simulink model "PulsePairProc"  (Simulink 6.4)
settings: Solver=ode45  StartTime=0.0  StopTime=40000/12e6  RelTol=1e-3
libraries: xbsIndex_r4 x256, simulink x2, dspsrcs4 x1
(part 1 of 2)
settings Model: LastModifiedBy=tbrimeye

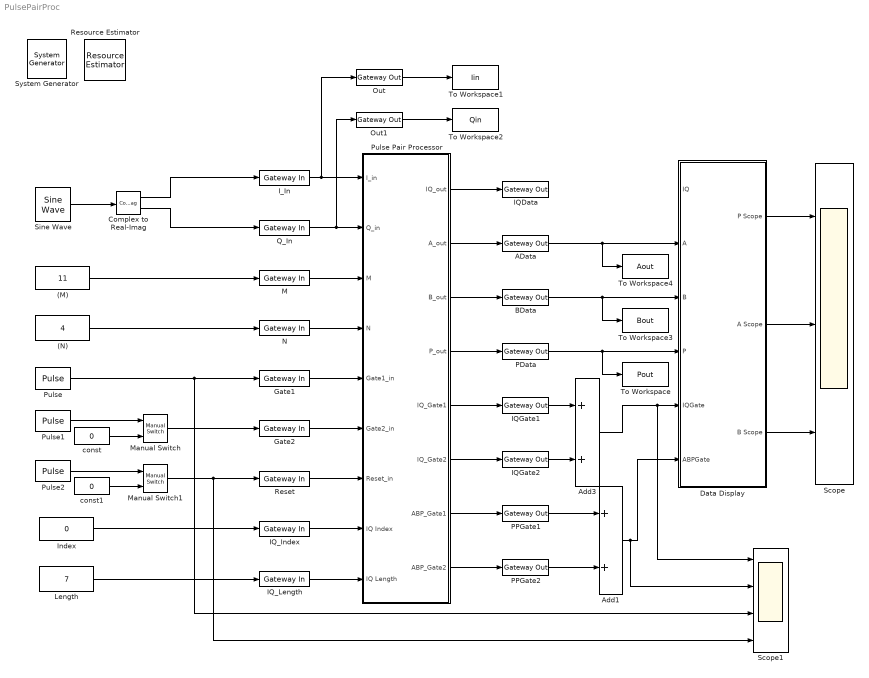
== system PulsePairProc ==
  " System Generator" : xbsIndex_r4/ System Generator  Tag=genX  SystemSampleTime=-1  xilinxfamily=Virtex4  part=xc4vlx60  speed=-11  package=ff668  synthesis_tool=XST  directory=C:/Work_Projects/Xilinx/SysGen_Outputs/PulsePairProcessor/PulsePairProc_x1_netlist  testbench=off  simulink_period=1/12e6  sysclk_period=(1/12e6)*1e9  incr_netlist=off  trim_vbits=Everywhere in SubSystem  dbl_ovrd=According to Block Masks  core_generation=According to Block Masks  run_coregen=off  deprecated_control=off  eval_field=0  block_type=sysgen
      settings: block_version=8.2
  (M) : Constant  Value=11  OutDataType=sfix(16)  ConRadixGroup=Use specified scaling  OutScaling=2^0  SampleTime=inf  FramePeriod=inf
  (N) : Constant  Value=4  OutDataType=sfix(16)  ConRadixGroup=Use specified scaling  OutScaling=2^0  SampleTime=inf  FramePeriod=inf
  AData : xbsIndex_r4/Gateway Out  hdl_port=on  timing_constraint=None  locs_specified=off  LOCs={}  block_type=gatewayout
      settings: infoedit="Gateway out block.  Converts Xilinx fixed point inputs into ouputs of type Simulink integer, double, or fixed point.<P><P>Hardware notes:  In hardware these blocks become top level output ports or are discarded, depending on how they are configured."  xl_area=[0 0 0 0 32 0 0]  block_version=8.2
  Add1 : Sum  OutScaling=2^-10
  Add3 : Sum  OutScaling=2^-10
  BData : xbsIndex_r4/Gateway Out  hdl_port=on  timing_constraint=None  locs_specified=off  LOCs={}  block_type=gatewayout
      settings: infoedit="Gateway out block.  Converts Xilinx fixed point inputs into ouputs of type Simulink integer, double, or fixed point.<P><P>Hardware notes:  In hardware these blocks become top level output ports or are discarded, depending on how they are configured."  xl_area=[0 0 0 0 32 0 0]  block_version=8.2
  Complex to Real-Imag : ComplexToRealImag
  Data Display : Subsystem
  Gate1 : xbsIndex_r4/Gateway In  arith_type=Boolean  n_bits=18  bin_pt=0  quantization="Round  (unbiased: +/- Inf)"  overflow=Flag as error  period=1/12e6  dbl_ovrd=off  timing_constraint=None  locs_specified=off  LOCs={}  block_type=gatewayin
      settings: infoedit="Gateway in block.  Converts inputs of type Simulink integer, double and fixed point to  Xilinx fixed point type.<P><P>Hardware notes:  In hardware these blocks become top level input ports."  xl_area=[0 0 0 0 1 0 0]  block_version=8.2
  Gate2 : xbsIndex_r4/Gateway In  arith_type=Boolean  n_bits=18  bin_pt=0  quantization="Round  (unbiased: +/- Inf)"  overflow=Flag as error  period=1/12e6  dbl_ovrd=off  timing_constraint=None  locs_specified=off  LOCs={}  block_type=gatewayin
      settings: infoedit="Gateway in block.  Converts inputs of type Simulink integer, double and fixed point to  Xilinx fixed point type.<P><P>Hardware notes:  In hardware these blocks become top level input ports."  xl_area=[0 0 0 0 1 0 0]  block_version=8.2
  IQData : xbsIndex_r4/Gateway Out  hdl_port=on  timing_constraint=None  locs_specified=off  LOCs={}  block_type=gatewayout
      settings: infoedit="Gateway out block.  Converts Xilinx fixed point inputs into ouputs of type Simulink integer, double, or fixed point.<P><P>Hardware notes:  In hardware these blocks become top level output ports or are discarded, depending on how they are configured."  xl_area=[0 0 0 0 32 0 0]  block_version=8.2
  IQGate1 : xbsIndex_r4/Gateway Out  hdl_port=on  timing_constraint=None  locs_specified=off  LOCs={}  block_type=gatewayout
      settings: infoedit="Gateway out block.  Converts Xilinx fixed point inputs into ouputs of type Simulink integer, double, or fixed point.<P><P>Hardware notes:  In hardware these blocks become top level output ports or are discarded, depending on how they are configured."  xl_area=[0 0 0 0 1 0 0]  block_version=8.2
  IQGate2 : xbsIndex_r4/Gateway Out  hdl_port=on  timing_constraint=None  locs_specified=off  LOCs={}  block_type=gatewayout
      settings: infoedit="Gateway out block.  Converts Xilinx fixed point inputs into ouputs of type Simulink integer, double, or fixed point.<P><P>Hardware notes:  In hardware these blocks become top level output ports or are discarded, depending on how they are configured."  xl_area=[0 0 0 0 1 0 0]  block_version=8.2
  IQ_Index : xbsIndex_r4/Gateway In  arith_type=Unsigned  n_bits=10  bin_pt=0  quantization="Round  (unbiased: +/- Inf)"  overflow=Flag as error  period=1/12e6  dbl_ovrd=off  timing_constraint=None  locs_specified=off  LOCs={}  block_type=gatewayin
      settings: infoedit="Gateway in block.  Converts inputs of type Simulink integer, double and fixed point to  Xilinx fixed point type.<P><P>Hardware notes:  In hardware these blocks become top level input ports."  xl_area=[0 0 0 0 10 0 0]  block_version=8.2
  IQ_Length : xbsIndex_r4/Gateway In  arith_type=Unsigned  n_bits=10  bin_pt=0  quantization="Round  (unbiased: +/- Inf)"  overflow=Flag as error  period=1/12e6  dbl_ovrd=off  timing_constraint=None  locs_specified=off  LOCs={}  block_type=gatewayin
      settings: infoedit="Gateway in block.  Converts inputs of type Simulink integer, double and fixed point to  Xilinx fixed point type.<P><P>Hardware notes:  In hardware these blocks become top level input ports."  xl_area=[0 0 0 0 10 0 0]  block_version=8.2
  I_In : xbsIndex_r4/Gateway In  arith_type="Signed  (2's comp)"  n_bits=16  bin_pt=15  quantization="Round  (unbiased: +/- Inf)"  overflow=Saturate  period=1/12e6  dbl_ovrd=off  timing_constraint=None  locs_specified=off  LOCs={}  block_type=gatewayin
      settings: infoedit="Gateway in block.  Converts inputs of type Simulink integer, double and fixed point to  Xilinx fixed point type.<P><P>Hardware notes:  In hardware these blocks become top level input ports."  xl_area=[0 0 0 0 16 0 0]  block_version=8.2
  Index : Constant  Value=0  OutDataType=sfix(16)  ConRadixGroup=Use specified scaling  OutScaling=2^0  SampleTime=inf  FramePeriod=inf
  Length : Constant  Value=7  OutDataType=sfix(16)  ConRadixGroup=Use specified scaling  OutScaling=2^0  SampleTime=inf  FramePeriod=inf
  M : xbsIndex_r4/Gateway In  arith_type=Unsigned  n_bits=11  bin_pt=0  quantization="Round  (unbiased: +/- Inf)"  overflow=Flag as error  period=1/12e6  dbl_ovrd=off  timing_constraint=None  locs_specified=off  LOCs={}  block_type=gatewayin
      settings: infoedit="Gateway in block.  Converts inputs of type Simulink integer, double and fixed point to  Xilinx fixed point type.<P><P>Hardware notes:  In hardware these blocks become top level input ports."  xl_area=[0 0 0 0 11 0 0]  block_version=8.2
  Manual Switch : simulink/Signal Routing/Manual Switch  SystemSampleTime=-1  sw=0  action=0
  Manual Switch1 : simulink/Signal Routing/Manual Switch  SystemSampleTime=-1  sw=1  action=0
  N : xbsIndex_r4/Gateway In  arith_type=Unsigned  n_bits=7  bin_pt=0  quantization="Round  (unbiased: +/- Inf)"  overflow=Flag as error  period=1/12e6  dbl_ovrd=off  timing_constraint=None  locs_specified=off  LOCs={}  block_type=gatewayin
      settings: infoedit="Gateway in block.  Converts inputs of type Simulink integer, double and fixed point to  Xilinx fixed point type.<P><P>Hardware notes:  In hardware these blocks become top level input ports."  xl_area=[0 0 0 0 7 0 0]  block_version=8.2
  Out : xbsIndex_r4/Gateway Out  hdl_port=off  timing_constraint=None  locs_specified=off  LOCs={}  block_type=gatewayout
      settings: infoedit="Gateway out block.  Converts Xilinx fixed point inputs into ouputs of type Simulink integer, double, or fixed point.<P><P>Hardware notes:  In hardware these blocks become top level output ports or are discarded, depending on how they are configured."  xl_area=[0 0 0 0 0 0 0]  block_version=8.2
  Out1 : xbsIndex_r4/Gateway Out  hdl_port=off  timing_constraint=None  locs_specified=off  LOCs={}  block_type=gatewayout
      settings: infoedit="Gateway out block.  Converts Xilinx fixed point inputs into ouputs of type Simulink integer, double, or fixed point.<P><P>Hardware notes:  In hardware these blocks become top level output ports or are discarded, depending on how they are configured."  xl_area=[0 0 0 0 0 0 0]  block_version=8.2
  PData : xbsIndex_r4/Gateway Out  hdl_port=on  timing_constraint=None  locs_specified=off  LOCs={}  block_type=gatewayout
      settings: infoedit="Gateway out block.  Converts Xilinx fixed point inputs into ouputs of type Simulink integer, double, or fixed point.<P><P>Hardware notes:  In hardware these blocks become top level output ports or are discarded, depending on how they are configured."  xl_area=[0 0 0 0 32 0 0]  block_version=8.2
  PPGate1 : xbsIndex_r4/Gateway Out  hdl_port=on  timing_constraint=None  locs_specified=off  LOCs={}  block_type=gatewayout
      settings: infoedit="Gateway out block.  Converts Xilinx fixed point inputs into ouputs of type Simulink integer, double, or fixed point.<P><P>Hardware notes:  In hardware these blocks become top level output ports or are discarded, depending on how they are configured."  xl_area=[0 0 0 0 1 0 0]  block_version=8.2
  PPGate2 : xbsIndex_r4/Gateway Out  hdl_port=on  timing_constraint=None  locs_specified=off  LOCs={}  block_type=gatewayout
      settings: infoedit="Gateway out block.  Converts Xilinx fixed point inputs into ouputs of type Simulink integer, double, or fixed point.<P><P>Hardware notes:  In hardware these blocks become top level output ports or are discarded, depending on how they are configured."  xl_area=[0 0 0 0 1 0 0]  block_version=8.2
  Pulse : DiscretePulseGenerator  PulseType=Time based  Period=22/12e6  PulseWidth=50  PhaseDelay=20/12e6
  Pulse Pair Processor : Subsystem
  Pulse1 : DiscretePulseGenerator  PulseType=Time based  Period=900/40e6  PulseWidth=10  PhaseDelay=150/12e6
  Pulse2 : DiscretePulseGenerator  PulseType=Time based  Period=500/12e6  PhaseDelay=10/12e6
  Q_In : xbsIndex_r4/Gateway In  arith_type="Signed  (2's comp)"  n_bits=16  bin_pt=15  quantization="Round  (unbiased: +/- Inf)"  overflow=Saturate  period=1/12e6  dbl_ovrd=off  timing_constraint=None  locs_specified=off  LOCs={}  block_type=gatewayin
      settings: infoedit="Gateway in block.  Converts inputs of type Simulink integer, double and fixed point to  Xilinx fixed point type.<P><P>Hardware notes:  In hardware these blocks become top level input ports."  xl_area=[0 0 0 0 16 0 0]  block_version=8.2
  Reset : xbsIndex_r4/Gateway In  arith_type=Boolean  n_bits=18  bin_pt=0  quantization="Round  (unbiased: +/- Inf)"  overflow=Flag as error  period=1/12e6  dbl_ovrd=off  timing_constraint=None  locs_specified=off  LOCs={}  block_type=gatewayin
      settings: infoedit="Gateway in block.  Converts inputs of type Simulink integer, double and fixed point to  Xilinx fixed point type.<P><P>Hardware notes:  In hardware these blocks become top level input ports."  xl_area=[0 0 0 0 1 0 0]  block_version=8.2
  Resource Estimator : xbsIndex_r4/Resource Estimator  Tag=resEstTag  Slices=1267  FFs=1392  BRAMs=16  LUTs=1882  IOBs=205  EBMs=6  TBUFs=0  xl_use_estimator_area=off  est_options=Post Map  xl_estimator_area=[1915 2342 0 3405 33 4 0]  block_type=resource_estimator
      settings: AttributesFormatString=Resource\nEstimator  block_version=8.2
  Scope : Scope  NumInputPorts=3
      settings: TimeRange=0.0035  YMin=0~-5~-5  YMax=5~5~5  MaxDataPoints=5000000
  Scope1 : Scope  NumInputPorts=4
      settings: TimeRange=0.0035  YMin=0~0~0~-5  YMax=2~2~2~5  MaxDataPoints=5000000
  Sine Wave : dspsrcs4/Sine Wave  Amplitude=.99  Frequency=100e3  Phase=0  SampleMode=Discrete  OutComplex=Complex  CompMethod=Trigonometric fcn  TableSize=Speed  SampleTime=1/12e6  SamplesPerFrame=1  dataType=double  wordLen=16  udDataType=sfix(16)  fracBitsMode=Best precision  numFracBits=15  ResetState=Restart at time zero
  To Workspace : ToWorkspace  VariableName=Pout  SampleTime=-1  SaveFormat=Array
  To Workspace1 : ToWorkspace  VariableName=Iin  SampleTime=-1  SaveFormat=Array
  To Workspace2 : ToWorkspace  VariableName=Qin  SampleTime=-1  SaveFormat=Array
  To Workspace3 : ToWorkspace  VariableName=Bout  SampleTime=-1  SaveFormat=Array
  To Workspace4 : ToWorkspace  VariableName=Aout  SampleTime=-1  SaveFormat=Array
  const : Constant  Value=0  OutDataType=sfix(16)  ConRadixGroup=Use specified scaling  OutScaling=2^0  SampleTime=inf  FramePeriod=inf
  const1 : Constant  Value=0  OutDataType=sfix(16)  ConRadixGroup=Use specified scaling  OutScaling=2^0  SampleTime=inf  FramePeriod=inf
  wires:
  I_In/1 -> Pulse Pair Processor/1(I_in), Out/1
  Q_In/1 -> Pulse Pair Processor/2(Q_in), Out1/1
  (M)/1 -> M/1
  (N)/1 -> N/1
  M/1 -> Pulse Pair Processor/3(M)
  N/1 -> Pulse Pair Processor/4(N)
  Pulse/1 -> Gate1/1, Scope1/3
  Pulse1/1 -> Manual Switch/1
  const/1 -> Manual Switch/2
  Manual Switch/1 -> Gate2/1
  Gate1/1 -> Pulse Pair Processor/5(Gate1_in)
  Gate2/1 -> Pulse Pair Processor/6(Gate2_in)
  Pulse Pair Processor/2(A_out) -> AData/1
  Pulse Pair Processor/3(B_out) -> BData/1
  Pulse Pair Processor/4(P_out) -> PData/1
  Data Display/1(P Scope) -> Scope/1
  Data Display/2(A Scope) -> Scope/2
  Data Display/3(B Scope) -> Scope/3
  Pulse Pair Processor/1(IQ_out) -> IQData/1
  Pulse Pair Processor/5(IQ_Gate1) -> IQGate1/1
  Pulse Pair Processor/6(IQ_Gate2) -> IQGate2/1
  IQGate1/1 -> Add3/1
  IQGate2/1 -> Add3/2
  Pulse Pair Processor/7(ABP_Gate1) -> PPGate1/1
  Pulse Pair Processor/8(ABP_Gate2) -> PPGate2/1
  PData/1 -> Data Display/4(P), To Workspace/1
  Reset/1 -> Pulse Pair Processor/7(Reset_in)
  Pulse2/1 -> Manual Switch1/1
  const1/1 -> Manual Switch1/2
  Manual Switch1/1 -> Reset/1, Scope1/4
  AData/1 -> Data Display/2(A), To Workspace4/1
  BData/1 -> Data Display/3(B), To Workspace3/1
  PPGate1/1 -> Add1/1
  PPGate2/1 -> Add1/2
  Add1/1 -> Data Display/6(ABPGate), Scope1/2
  Sine Wave/1 -> Complex to Real-Imag/1
  Complex to Real-Imag/1 -> I_In/1
  Complex to Real-Imag/2 -> Q_In/1
  Add3/1 -> Data Display/5(IQGate), Scope1/1
  IQ_Index/1 -> Pulse Pair Processor/8(IQ Index)
  IQ_Length/1 -> Pulse Pair Processor/9(IQ Length)
  Index/1 -> IQ_Index/1
  Length/1 -> IQ_Length/1
  Out/1 -> To Workspace1/1
  Out1/1 -> To Workspace2/1

== system PulsePairProc/Data Display ==
  IQ : Inport
  A : Inport  Port=2
  B : Inport  Port=3
  P : Inport  Port=4
  IQGate : Inport  Port=5
  ABPGate : Inport  Port=6
  Mux : Mux
  Mux1 : Mux
  Mux2 : Mux
  P Scope : Outport
  A Scope : Outport  Port=2
  B Scope : Outport  Port=3
  wires:
  IQ/1 -> Mux/1, Mux1/1, Mux2/1
  Mux/1 -> P Scope/1
  Mux1/1 -> A Scope/1
  Mux2/1 -> B Scope/1
  P/1 -> Mux/2
  IQGate/1 -> Mux1/2, Mux2/2, Mux/3
  ABPGate/1 -> Mux1/4, Mux2/4, Mux/4
  A/1 -> Mux1/3
  B/1 -> Mux2/3

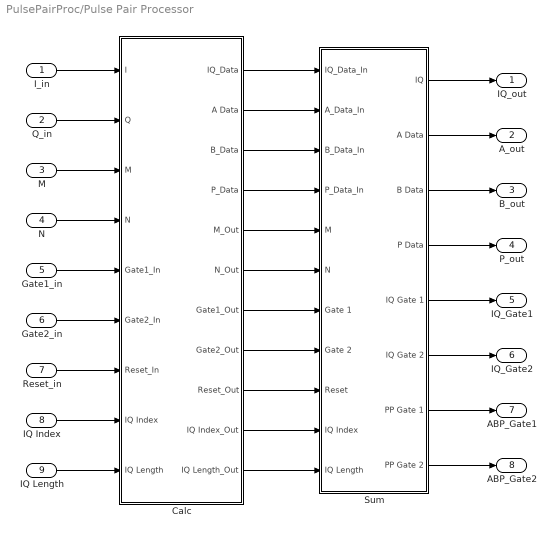
== system PulsePairProc/Pulse Pair Processor ==
  I_in : Inport
  Q_in : Inport  Port=2
  M : Inport  Port=3
  N : Inport  Port=4
  Gate1_in : Inport  Port=5
  Gate2_in : Inport  Port=6
  Reset_in : Inport  Port=7
  IQ Index : Inport  Port=8
  IQ Length : Inport  Port=9
  Calc : Subsystem
  Sum : Subsystem
  IQ_out : Outport
  A_out : Outport  Port=2
  B_out : Outport  Port=3
  P_out : Outport  Port=4
  IQ_Gate1 : Outport  Port=5
  IQ_Gate2 : Outport  Port=6
  ABP_Gate1 : Outport  Port=7
  ABP_Gate2 : Outport  Port=8
  wires:
  Calc/2(A Data) -> Sum/2(A_Data_In)
  Calc/3(B_Data) -> Sum/3(B_Data_In)
  Calc/4(P_Data) -> Sum/4(P_Data_In)
  Calc/5(M_Out) -> Sum/5(M)
  Calc/6(N_Out) -> Sum/6(N)
  Calc/7(Gate1_Out) -> Sum/7(Gate 1)
  Calc/8(Gate2_Out) -> Sum/8(Gate 2)
  Calc/1(IQ_Data) -> Sum/1(IQ_Data_In)
  Calc/9(Reset_Out) -> Sum/9(Reset)
  Sum/1(IQ) -> IQ_out/1
  I_in/1 -> Calc/1(I)
  Q_in/1 -> Calc/2(Q)
  M/1 -> Calc/3(M)
  N/1 -> Calc/4(N)
  Gate1_in/1 -> Calc/5(Gate1_In)
  Sum/5(IQ Gate 1) -> IQ_Gate1/1
  Sum/6(IQ Gate 2) -> IQ_Gate2/1
  Gate2_in/1 -> Calc/6(Gate2_In)
  Sum/7(PP Gate 1) -> ABP_Gate1/1
  Reset_in/1 -> Calc/7(Reset_In)
  Sum/8(PP Gate 2) -> ABP_Gate2/1
  Sum/2(A Data) -> A_out/1
  Sum/3(B Data) -> B_out/1
  Sum/4(P Data) -> P_out/1
  IQ Index/1 -> Calc/8(IQ Index)
  IQ Length/1 -> Calc/9(IQ Length)
  Calc/10(IQ Index_Out) -> Sum/10(IQ Index)
  Calc/11(IQ Length_Out) -> Sum/11(IQ Length)

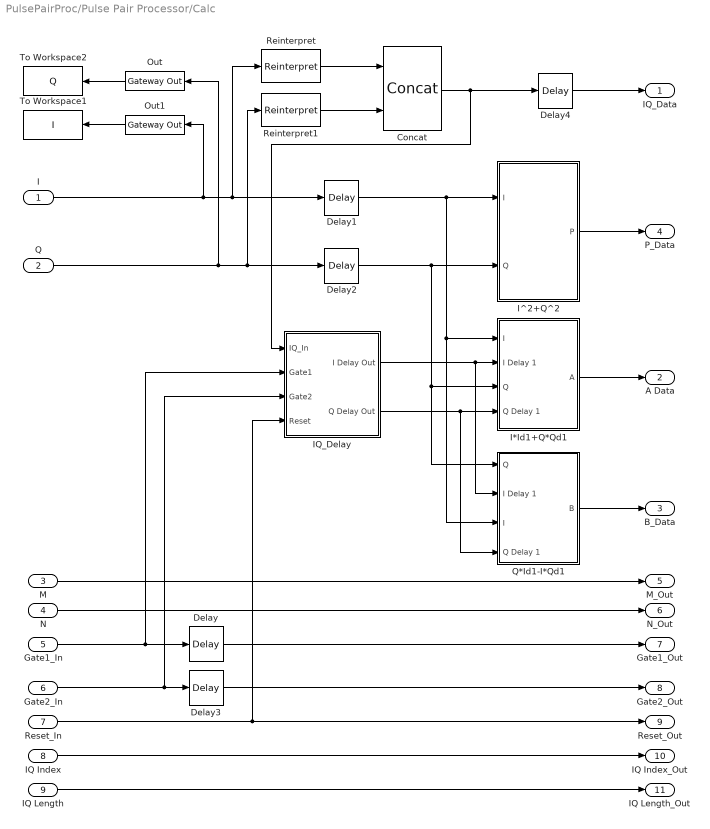
== system PulsePairProc/Pulse Pair Processor/Calc ==
  I : Inport
  Q : Inport  Port=2
  M : Inport  Port=3
  N : Inport  Port=4
  Gate1_In : Inport  Port=5
  Gate2_In : Inport  Port=6
  Reset_In : Inport  Port=7
  IQ Index : Inport  Port=8
  IQ Length : Inport  Port=9
  Concat : xbsIndex_r4/Concat  num_inputs=2  dbl_ovrd=off  block_type=concat
      settings: block_version=8.2
  Delay : xbsIndex_r4/Delay  en=off  latency=6  dbl_ovrd=off  reg_retiming=off  block_type=delay
      settings: infoedit=Hardware notes: A delay line is a chain, each link of which is an SRL16 followed by a flip-flop. If register retiming is enabled, the delay line is a chain of flip-flops.  block_version=8.2
  Delay1 : xbsIndex_r4/Delay  en=off  latency=4  dbl_ovrd=off  reg_retiming=off  block_type=delay
      settings: infoedit=Hardware notes: A delay line is a chain, each link of which is an SRL16 followed by a flip-flop. If register retiming is enabled, the delay line is a chain of flip-flops.  block_version=8.2
  Delay2 : xbsIndex_r4/Delay  en=off  latency=4  dbl_ovrd=off  reg_retiming=off  block_type=delay
      settings: infoedit=Hardware notes: A delay line is a chain, each link of which is an SRL16 followed by a flip-flop. If register retiming is enabled, the delay line is a chain of flip-flops.  block_version=8.2
  Delay3 : xbsIndex_r4/Delay  en=off  latency=6  dbl_ovrd=off  reg_retiming=off  block_type=delay
      settings: infoedit=Hardware notes: A delay line is a chain, each link of which is an SRL16 followed by a flip-flop. If register retiming is enabled, the delay line is a chain of flip-flops.  block_version=8.2
  Delay4 : xbsIndex_r4/Delay  en=off  latency=6  dbl_ovrd=off  reg_retiming=off  block_type=delay
      settings: infoedit=Hardware notes: A delay line is a chain, each link of which is an SRL16 followed by a flip-flop. If register retiming is enabled, the delay line is a chain of flip-flops.  block_version=8.2
  I*Id1+Q*Qd1 : Subsystem
  IQ_Delay : Subsystem
  I^2+Q^2 : Subsystem
  Out : xbsIndex_r4/Gateway Out  Orientation=left  hdl_port=off  timing_constraint=None  locs_specified=off  LOCs={}  block_type=gatewayout
      settings: infoedit="Gateway out block.  Converts Xilinx fixed point inputs into ouputs of type Simulink integer, double, or fixed point.<P><P>Hardware notes:  In hardware these blocks become top level output ports or are discarded, depending on how they are configured."  xl_area=[0 0 0 0 0 0 0]  block_version=8.2
  Out1 : xbsIndex_r4/Gateway Out  Orientation=left  hdl_port=off  timing_constraint=None  locs_specified=off  LOCs={}  block_type=gatewayout
      settings: infoedit="Gateway out block.  Converts Xilinx fixed point inputs into ouputs of type Simulink integer, double, or fixed point.<P><P>Hardware notes:  In hardware these blocks become top level output ports or are discarded, depending on how they are configured."  xl_area=[0 0 0 0 0 0 0]  block_version=8.2
  Q*Id1-I*Qd1 : Subsystem
  Reinterpret : xbsIndex_r4/Reinterpret  force_arith_type=on  arith_type=Unsigned  force_bin_pt=on  bin_pt=0  block_type=reinterpret
      settings: infoedit="Changes signal type without altering the binary representation.   You can changed the signal between signed and unsigned, and relocate the binary point.<P><P>Hardware notes: In hardware this block costs nothing.<P><P>Example:  Suppose the input is 6 bits wide, signed, with 2 fractional bits, and the output is forced to unsigned with 0 fractional bits.  Then an input of -2.0 (1110.00 in binary 2's complement) becomes an output of 56 (111000 in binary)."  block_version=8.2
  Reinterpret1 : xbsIndex_r4/Reinterpret  force_arith_type=on  arith_type=Unsigned  force_bin_pt=on  bin_pt=0  block_type=reinterpret
      settings: infoedit="Changes signal type without altering the binary representation.   You can changed the signal between signed and unsigned, and relocate the binary point.<P><P>Hardware notes: In hardware this block costs nothing.<P><P>Example:  Suppose the input is 6 bits wide, signed, with 2 fractional bits, and the output is forced to unsigned with 0 fractional bits.  Then an input of -2.0 (1110.00 in binary 2's complement) becomes an output of 56 (111000 in binary)."  block_version=8.2
  To Workspace1 : ToWorkspace  VariableName=I  SampleTime=-1  SaveFormat=Array
  To Workspace2 : ToWorkspace  VariableName=Q  SampleTime=-1  SaveFormat=Array
  IQ_Data : Outport
  A Data : Outport  Port=2
  B_Data : Outport  Port=3
  P_Data : Outport  Port=4
  M_Out : Outport  Port=5
  N_Out : Outport  Port=6
  Gate1_Out : Outport  Port=7
  Gate2_Out : Outport  Port=8
  Reset_Out : Outport  Port=9
  IQ Index_Out : Outport  Port=10
  IQ Length_Out : Outport  Port=11
  wires:
  Gate1_In/1 -> Delay/1, IQ_Delay/2(Gate1)
  Gate2_In/1 -> Delay3/1, IQ_Delay/3(Gate2)
  I^2+Q^2/1(P) -> P_Data/1
  I*Id1+Q*Qd1/1(A) -> A Data/1
  Q*Id1-I*Qd1/1(B) -> B_Data/1
  Delay/1 -> Gate1_Out/1
  Delay3/1 -> Gate2_Out/1
  M/1 -> M_Out/1
  N/1 -> N_Out/1
  Concat/1 -> Delay4/1, IQ_Delay/1(IQ_In)
  Reinterpret/1 -> Concat/1
  Reinterpret1/1 -> Concat/2
  Reset_In/1 -> Reset_Out/1, IQ_Delay/4(Reset)
  Delay1/1 -> I*Id1+Q*Qd1/1(I), Q*Id1-I*Qd1/3(I), I^2+Q^2/1(I)
  Delay2/1 -> I*Id1+Q*Qd1/3(Q), Q*Id1-I*Qd1/1(Q), I^2+Q^2/2(Q)
  IQ_Delay/1(I Delay Out) -> I*Id1+Q*Qd1/2(I Delay 1), Q*Id1-I*Qd1/2(I Delay 1)
  IQ_Delay/2(Q Delay Out) -> I*Id1+Q*Qd1/4(Q Delay 1), Q*Id1-I*Qd1/4(Q Delay 1)
  Delay4/1 -> IQ_Data/1
  IQ Index/1 -> IQ Index_Out/1
  IQ Length/1 -> IQ Length_Out/1
  I/1 -> Reinterpret/1, Delay1/1, Out1/1
  Q/1 -> Delay2/1, Reinterpret1/1, Out/1
  Out/1 -> To Workspace2/1
  Out1/1 -> To Workspace1/1

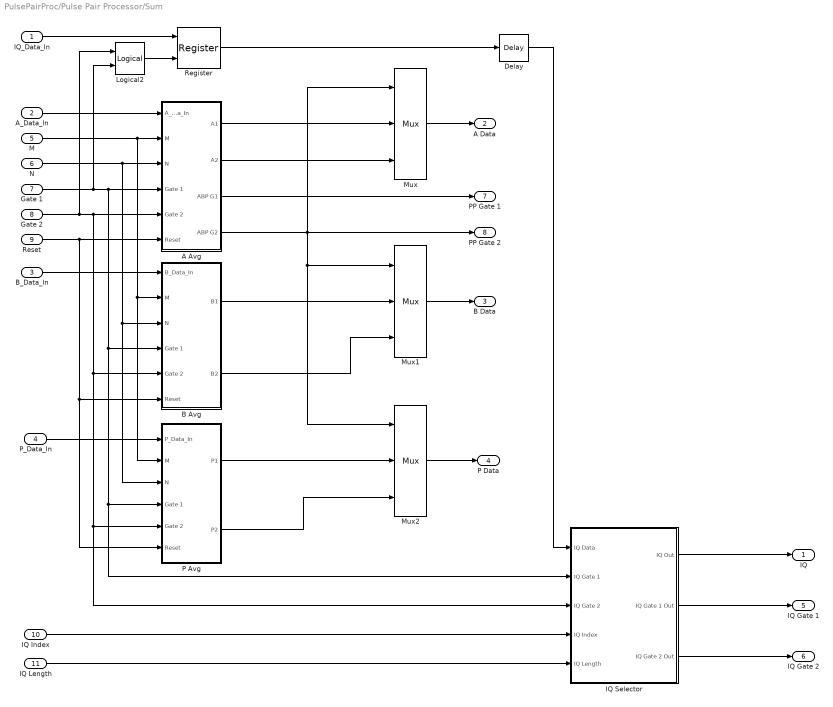
== system PulsePairProc/Pulse Pair Processor/Sum ==
  IQ_Data_In : Inport
  A_Data_In : Inport  Port=2
  B_Data_In : Inport  Port=3
  P_Data_In : Inport  Port=4
  M : Inport  Port=5
  N : Inport  Port=6
  Gate 1 : Inport  Port=7
  Gate 2 : Inport  Port=8
  Reset : Inport  Port=9
  IQ Index : Inport  Port=10
  IQ Length : Inport  Port=11
  A Avg : Subsystem
  B Avg : Subsystem
  Delay : xbsIndex_r4/Delay  en=off  latency=2  dbl_ovrd=off  reg_retiming=off  block_type=delay
      settings: infoedit=Hardware notes: A delay line is a chain, each link of which is an SRL16 followed by a flip-flop. If register retiming is enabled, the delay line is a chain of flip-flops.  block_version=8.2
  IQ Selector : Subsystem
  Logical2 : xbsIndex_r4/Logical  logical_function=NOR  inputs=2  en=off  latency=0  precision=Full  arith_type=Unsigned  n_bits=16  bin_pt=0  align_bp=on  dbl_ovrd=off  block_type=logical
      settings: block_version=8.2
  Mux : xbsIndex_r4/Mux  inputs=2  en=off  latency=0  precision=Full  arith_type=Unsigned  n_bits=16  bin_pt=14  quantization=Truncate  overflow=Wrap  dbl_ovrd=off  block_type=mux
      settings: block_version=8.2
  Mux1 : xbsIndex_r4/Mux  inputs=2  en=off  latency=0  precision=Full  arith_type=Unsigned  n_bits=16  bin_pt=14  quantization=Truncate  overflow=Wrap  dbl_ovrd=off  block_type=mux
      settings: block_version=8.2
  Mux2 : xbsIndex_r4/Mux  inputs=2  en=off  latency=0  precision=Full  arith_type=Unsigned  n_bits=16  bin_pt=14  quantization=Truncate  overflow=Wrap  dbl_ovrd=off  block_type=mux
      settings: block_version=8.2
  P Avg : Subsystem
  Register : xbsIndex_r4/Register  init=0  rst=on  en=off  dbl_ovrd=off  block_type=register
      settings: block_version=8.2
  IQ : Outport
  A Data : Outport  Port=2
  B Data : Outport  Port=3
  P Data : Outport  Port=4
  IQ Gate 1 : Outport  Port=5
  IQ Gate 2 : Outport  Port=6
  PP Gate 1 : Outport  Port=7
  PP Gate 2 : Outport  Port=8
  wires:
  A_Data_In/1 -> A Avg/1(A_Data_In)
  M/1 -> A Avg/2(M), B Avg/2(M), P Avg/2(M)
  N/1 -> A Avg/3(N), B Avg/3(N), P Avg/3(N)
  Gate 1/1 -> A Avg/4(Gate 1), B Avg/4(Gate 1), P Avg/4(Gate 1), IQ Selector/2(IQ Gate 1), Logical2/2
  Gate 2/1 -> A Avg/5(Gate 2), B Avg/5(Gate 2), P Avg/5(Gate 2), IQ Selector/3(IQ Gate 2), Logical2/1
  B_Data_In/1 -> B Avg/1(B_Data_In)
  P_Data_In/1 -> P Avg/1(P_Data_In)
  A Avg/3(ABP G1) -> PP Gate 1/1
  A Avg/4(ABP G2) -> PP Gate 2/1, Mux/1, Mux1/1, Mux2/1
  Reset/1 -> A Avg/6(Reset), B Avg/6(Reset), P Avg/6(Reset)
  IQ_Data_In/1 -> Register/1
  Logical2/1 -> Register/2
  Mux/1 -> A Data/1
  A Avg/1(A1) -> Mux/2
  A Avg/2(A2) -> Mux/3
  Mux1/1 -> B Data/1
  B Avg/1(B1) -> Mux1/2
  B Avg/2(B2) -> Mux1/3
  Mux2/1 -> P Data/1
  P Avg/1(P1) -> Mux2/2
  P Avg/2(P2) -> Mux2/3
  IQ Selector/1(IQ Out) -> IQ/1
  IQ Index/1 -> IQ Selector/4(IQ Index)
  IQ Length/1 -> IQ Selector/5(IQ Length)
  IQ Selector/2(IQ Gate 1 Out) -> IQ Gate 1/1
  IQ Selector/3(IQ Gate 2 Out) -> IQ Gate 2/1
  Register/1 -> Delay/1
  Delay/1 -> IQ Selector/1(IQ Data)

== system PulsePairProc/Pulse Pair Processor/Calc/I*Id1+Q*Qd1 ==
  I : Inport
  I Delay 1 : Inport  Port=2
  Q : Inport  Port=3
  Q Delay 1 : Inport  Port=4
  AddSub1 : xbsIndex_r4/AddSub  mode=Addition  use_carryin=off  use_carryout=off  en=off  latency=1  precision=User Defined  arith_type="Signed  (2's comp)"  n_bits=32  bin_pt=31  quantization="Round  (unbiased: +/- Inf)"  overflow=Flag as error  dbl_ovrd=off  use_behavioral_HDL=off  pipelined=on  use_rpm=on  block_type=addsub
      settings: block_version=8.2
  Mult2 : xbsIndex_r4/Mult  precision=User Defined  arith_type="Signed  (2's comp)"  n_bits=32  bin_pt=31  quantization="Round  (unbiased: +/- Inf)"  overflow=Saturate  en=off  latency=1  dbl_ovrd=off  use_behavioral_HDL=off  use_embedded=on  optimum_pipeline=off  use_rpm=on  placement_style=Rectangular shape  pipeline=on  block_type=mult
      settings: infoedit=Hardware notes: To use the internal pipeline stage of the dedicated multiplier you must select 'Pipeline for maximum performance'.  block_version=8.2
  Mult3 : xbsIndex_r4/Mult  precision=User Defined  arith_type="Signed  (2's comp)"  n_bits=32  bin_pt=31  quantization="Round  (unbiased: +/- Inf)"  overflow=Saturate  en=off  latency=1  dbl_ovrd=off  use_behavioral_HDL=off  use_embedded=on  optimum_pipeline=off  use_rpm=on  placement_style=Rectangular shape  pipeline=on  block_type=mult
      settings: infoedit=Hardware notes: To use the internal pipeline stage of the dedicated multiplier you must select 'Pipeline for maximum performance'.  block_version=8.2
  A : Outport
  wires:
  Mult2/1 -> AddSub1/1
  Mult3/1 -> AddSub1/2
  I/1 -> Mult2/1
  I Delay 1/1 -> Mult2/2
  AddSub1/1 -> A/1
  Q/1 -> Mult3/1
  Q Delay 1/1 -> Mult3/2

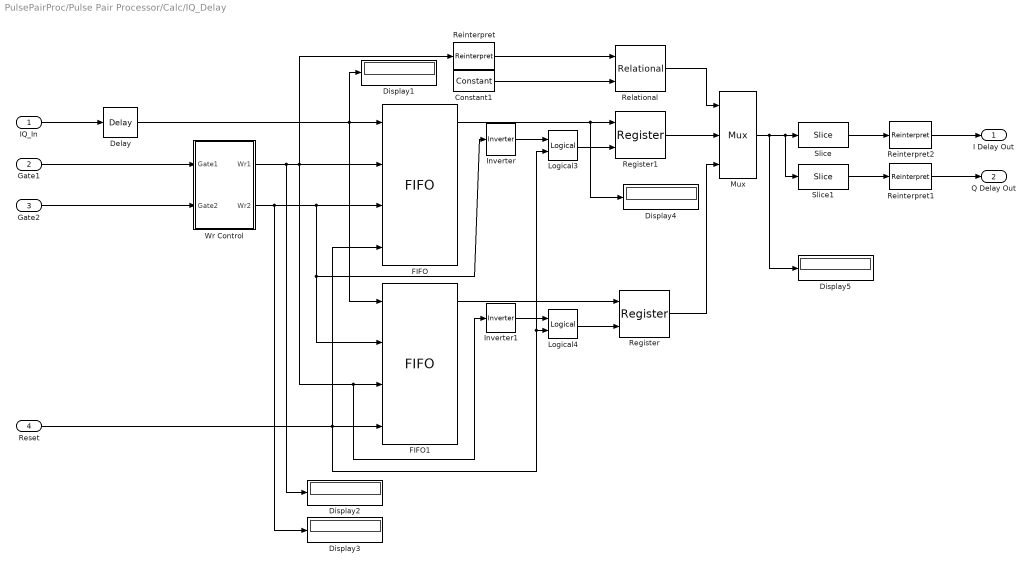
== system PulsePairProc/Pulse Pair Processor/Calc/IQ_Delay ==
  IQ_In : Inport
  Gate1 : Inport  Port=2
  Gate2 : Inport  Port=3
  Reset : Inport  Port=4
  Constant1 : xbsIndex_r4/Constant  arith_type=Unsigned  const=1  n_bits=1  bin_pt=0  explicit_period=off  period=1  equ=P=C  opselect=C  inp2=PCIN>>17  opr=+  inp1=P  carry=CIN  dbl_ovrd=off  block_type=constant
      settings: block_version=8.2
  Delay : xbsIndex_r4/Delay  en=off  latency=2  dbl_ovrd=off  reg_retiming=off  block_type=delay
      settings: infoedit=Hardware notes: A delay line is a chain, each link of which is an SRL16 followed by a flip-flop. If register retiming is enabled, the delay line is a chain of flip-flops.  block_version=8.2
  Display{1..5} (5 alike) : Display
  FIFO : xbsIndex_r4/FIFO  depth=1K  percent_nbits=1  rst=on  en=off  dbl_ovrd=off  mem_type=Block RAM  block_type=fifo
      settings: block_version=8.2
  FIFO1 : xbsIndex_r4/FIFO  depth=1K  percent_nbits=1  rst=on  en=off  dbl_ovrd=off  mem_type=Block RAM  block_type=fifo
      settings: block_version=8.2
  Inverter : xbsIndex_r4/Inverter  en=off  latency=1  dbl_ovrd=off  block_type=inv
      settings: block_version=8.2
  Inverter1 : xbsIndex_r4/Inverter  en=off  latency=1  dbl_ovrd=off  block_type=inv
      settings: block_version=8.2
  Logical3 : xbsIndex_r4/Logical  logical_function=OR  inputs=2  en=off  latency=0  precision=Full  arith_type=Unsigned  n_bits=16  bin_pt=0  align_bp=on  dbl_ovrd=off  block_type=logical
      settings: block_version=8.2
  Logical4 : xbsIndex_r4/Logical  logical_function=OR  inputs=2  en=off  latency=0  precision=Full  arith_type=Unsigned  n_bits=16  bin_pt=0  align_bp=on  dbl_ovrd=off  block_type=logical
      settings: block_version=8.2
  Mux : xbsIndex_r4/Mux  inputs=2  en=off  latency=0  precision=Full  arith_type=Unsigned  n_bits=16  bin_pt=14  quantization=Truncate  overflow=Wrap  dbl_ovrd=off  block_type=mux
      settings: block_version=8.2
  Register : xbsIndex_r4/Register  init=0  rst=on  en=off  dbl_ovrd=off  block_type=register
      settings: block_version=8.2
  Register1 : xbsIndex_r4/Register  init=0  rst=on  en=off  dbl_ovrd=off  block_type=register
      settings: block_version=8.2
  Reinterpret : xbsIndex_r4/Reinterpret  force_arith_type=on  arith_type=Unsigned  force_bin_pt=off  bin_pt=0  block_type=reinterpret
      settings: infoedit="Changes signal type without altering the binary representation.   You can changed the signal between signed and unsigned, and relocate the binary point.<P><P>Hardware notes: In hardware this block costs nothing.<P><P>Example:  Suppose the input is 6 bits wide, signed, with 2 fractional bits, and the output is forced to unsigned with 0 fractional bits.  Then an input of -2.0 (1110.00 in binary 2's complement) becomes an output of 56 (111000 in binary)."  block_version=8.2
  Reinterpret1 : xbsIndex_r4/Reinterpret  force_arith_type=on  arith_type="Signed  (2's comp)"  force_bin_pt=on  bin_pt=15  block_type=reinterpret
      settings: infoedit="Changes signal type without altering the binary representation.   You can changed the signal between signed and unsigned, and relocate the binary point.<P><P>Hardware notes: In hardware this block costs nothing.<P><P>Example:  Suppose the input is 6 bits wide, signed, with 2 fractional bits, and the output is forced to unsigned with 0 fractional bits.  Then an input of -2.0 (1110.00 in binary 2's complement) becomes an output of 56 (111000 in binary)."  block_version=8.2
  Reinterpret2 : xbsIndex_r4/Reinterpret  force_arith_type=on  arith_type="Signed  (2's comp)"  force_bin_pt=on  bin_pt=15  block_type=reinterpret
      settings: infoedit="Changes signal type without altering the binary representation.   You can changed the signal between signed and unsigned, and relocate the binary point.<P><P>Hardware notes: In hardware this block costs nothing.<P><P>Example:  Suppose the input is 6 bits wide, signed, with 2 fractional bits, and the output is forced to unsigned with 0 fractional bits.  Then an input of -2.0 (1110.00 in binary 2's complement) becomes an output of 56 (111000 in binary)."  block_version=8.2
  Relational : xbsIndex_r4/Relational  mode=a=b  en=off  latency=2  dbl_ovrd=off  block_type=relational
      settings: block_version=8.2
  Slice : xbsIndex_r4/Slice  nbits=16  boolean_output=off  mode=Upper Bit Location + Width  bit1=0  base1=MSB of Input  bit0=0  base0=LSB of Input  dbl_ovrd=off  block_type=slice
      settings: infoedit="Extracts a given range of bits from each input sample and presents it at the output.  The output type is ordinarily unsigned with binary point at zero, but can be Boolean when the slice is one bit wide.<P><P>Hardware notes: In hardware this block costs nothing."  block_version=8.2
  Slice1 : xbsIndex_r4/Slice  nbits=16  boolean_output=off  mode=Lower Bit Location + Width  bit1=0  base1=MSB of Input  bit0=0  base0=LSB of Input  dbl_ovrd=off  block_type=slice
      settings: infoedit="Extracts a given range of bits from each input sample and presents it at the output.  The output type is ordinarily unsigned with binary point at zero, but can be Boolean when the slice is one bit wide.<P><P>Hardware notes: In hardware this block costs nothing."  block_version=8.2
  Wr Control : Subsystem
  I Delay Out : Outport
  Q Delay Out : Outport  Port=2
  wires:
  IQ_In/1 -> Delay/1
  Reset/1 -> FIFO/4, FIFO1/4, Logical4/2, Logical3/2
  FIFO1/1 -> Register/1
  FIFO/1 -> Register1/1, Display4/1
  Register1/1 -> Mux/2
  Register/1 -> Mux/3
  Relational/1 -> Mux/1
  Constant1/1 -> Relational/2
  Reinterpret/1 -> Relational/1
  Delay/1 -> FIFO1/1, FIFO/1, Display1/1
  Logical3/1 -> Register1/2
  Logical4/1 -> Register/2
  Inverter1/1 -> Logical4/1
  Inverter/1 -> Logical3/1
  Mux/1 -> Slice/1, Slice1/1, Display5/1
  Slice/1 -> Reinterpret2/1
  Slice1/1 -> Reinterpret1/1
  Reinterpret1/1 -> Q Delay Out/1
  Reinterpret2/1 -> I Delay Out/1
  Wr Control/1(Wr1) -> FIFO/2, Reinterpret/1, FIFO1/3, Inverter1/1, Display2/1
  Wr Control/2(Wr2) -> FIFO/3, FIFO1/2, Inverter/1, Display3/1
  Gate1/1 -> Wr Control/1(Gate1)
  Gate2/1 -> Wr Control/2(Gate2)

== system PulsePairProc/Pulse Pair Processor/Calc/I^2+Q^2 ==
  I : Inport
  Q : Inport  Port=2
  AddSub : xbsIndex_r4/AddSub  mode=Addition  use_carryin=off  use_carryout=off  en=off  latency=1  precision=User Defined  arith_type=Unsigned  n_bits=32  bin_pt=32  quantization="Round  (unbiased: +/- Inf)"  overflow=Flag as error  dbl_ovrd=off  use_behavioral_HDL=off  pipelined=on  use_rpm=on  block_type=addsub
      settings: block_version=8.2
  Mult : xbsIndex_r4/Mult  precision=User Defined  arith_type=Unsigned  n_bits=32  bin_pt=32  quantization="Round  (unbiased: +/- Inf)"  overflow=Flag as error  en=off  latency=1  dbl_ovrd=off  use_behavioral_HDL=off  use_embedded=on  optimum_pipeline=off  use_rpm=on  placement_style=Rectangular shape  pipeline=on  block_type=mult
      settings: infoedit=Hardware notes: To use the internal pipeline stage of the dedicated multiplier you must select 'Pipeline for maximum performance'.  block_version=8.2
  Mult1 : xbsIndex_r4/Mult  precision=User Defined  arith_type=Unsigned  n_bits=32  bin_pt=32  quantization="Round  (unbiased: +/- Inf)"  overflow=Flag as error  en=off  latency=1  dbl_ovrd=off  use_behavioral_HDL=off  use_embedded=on  optimum_pipeline=off  use_rpm=on  placement_style=Rectangular shape  pipeline=on  block_type=mult
      settings: infoedit=Hardware notes: To use the internal pipeline stage of the dedicated multiplier you must select 'Pipeline for maximum performance'.  block_version=8.2
  To Workspace1 : ToWorkspace  VariableName=Isq  SampleTime=-1  SaveFormat=Array
  To Workspace2 : ToWorkspace  VariableName=Qsq  SampleTime=-1  SaveFormat=Array
  To Workspace3 : ToWorkspace  VariableName=Ppp  SampleTime=-1  SaveFormat=Array
  P : Outport
  wires:
  Mult/1 -> To Workspace1/1, AddSub/1
  Mult1/1 -> To Workspace2/1, AddSub/2
  I/1 -> Mult/1, Mult/2
  Q/1 -> Mult1/1, Mult1/2
  AddSub/1 -> P/1, To Workspace3/1

== system PulsePairProc/Pulse Pair Processor/Calc/Q*Id1-I*Qd1 ==
  Q : Inport
  I Delay 1 : Inport  Port=2
  I : Inport  Port=3
  Q Delay 1 : Inport  Port=4
  AddSub2 : xbsIndex_r4/AddSub  mode=Subtraction  use_carryin=off  use_carryout=off  en=off  latency=1  precision=User Defined  arith_type="Signed  (2's comp)"  n_bits=32  bin_pt=31  quantization="Round  (unbiased: +/- Inf)"  overflow=Flag as error  dbl_ovrd=off  use_behavioral_HDL=off  pipelined=on  use_rpm=on  block_type=addsub
      settings: block_version=8.2
  Mult4 : xbsIndex_r4/Mult  precision=User Defined  arith_type="Signed  (2's comp)"  n_bits=32  bin_pt=31  quantization="Round  (unbiased: +/- Inf)"  overflow=Saturate  en=off  latency=1  dbl_ovrd=off  use_behavioral_HDL=off  use_embedded=on  optimum_pipeline=off  use_rpm=on  placement_style=Rectangular shape  pipeline=on  block_type=mult
      settings: infoedit=Hardware notes: To use the internal pipeline stage of the dedicated multiplier you must select 'Pipeline for maximum performance'.  block_version=8.2
  Mult5 : xbsIndex_r4/Mult  precision=User Defined  arith_type="Signed  (2's comp)"  n_bits=32  bin_pt=31  quantization="Round  (unbiased: +/- Inf)"  overflow=Saturate  en=off  latency=1  dbl_ovrd=off  use_behavioral_HDL=off  use_embedded=on  optimum_pipeline=off  use_rpm=on  placement_style=Rectangular shape  pipeline=on  block_type=mult
      settings: infoedit=Hardware notes: To use the internal pipeline stage of the dedicated multiplier you must select 'Pipeline for maximum performance'.  block_version=8.2
  B : Outport
  wires:
  Mult4/1 -> AddSub2/1
  Mult5/1 -> AddSub2/2
  Q/1 -> Mult4/1
  I Delay 1/1 -> Mult4/2
  AddSub2/1 -> B/1
  I/1 -> Mult5/1
  Q Delay 1/1 -> Mult5/2

== system PulsePairProc/Pulse Pair Processor/Sum/A Avg ==
  A_Data_In : Inport
  M : Inport  Port=2
  N : Inport  Port=3
  Gate 1 : Inport  Port=4
  Gate 2 : Inport  Port=5
  Reset : Inport  Port=6
  Avg. A 1 : Subsystem
  Avg. A 2 : Subsystem
  A1 : Outport
  A2 : Outport  Port=2
  ABP G1 : Outport  Port=3
  ABP G2 : Outport  Port=4
  wires:
  A_Data_In/1 -> Avg. A 1/1(In), Avg. A 2/1(In)
  M/1 -> Avg. A 1/2(M), Avg. A 2/2(M)
  N/1 -> Avg. A 1/3(N), Avg. A 2/3(N)
  Avg. A 1/1(Out) -> A1/1
  Gate 1/1 -> Avg. A 1/4(Gate)
  Avg. A 2/1(Out) -> A2/1
  Gate 2/1 -> Avg. A 2/4(Gate)
  Avg. A 1/2(A,B,P Gate 1) -> ABP G1/1
  Avg. A 2/2(A,B,P Gate 1) -> ABP G2/1
  Reset/1 -> Avg. A 1/5(Reset), Avg. A 2/5(Reset)

== system PulsePairProc/Pulse Pair Processor/Sum/B Avg ==
  B_Data_In : Inport
  M : Inport  Port=2
  N : Inport  Port=3
  Gate 1 : Inport  Port=4
  Gate 2 : Inport  Port=5
  Reset : Inport  Port=6
  Avg. B 1 : Subsystem
  Avg. B 2 : Subsystem
  B1 : Outport
  B2 : Outport  Port=2
  wires:
  B_Data_In/1 -> Avg. B 1/1(In), Avg. B 2/1(In)
  M/1 -> Avg. B 1/2(M), Avg. B 2/2(M)
  N/1 -> Avg. B 1/3(N), Avg. B 2/3(N)
  Avg. B 1/1(Out) -> B1/1
  Gate 1/1 -> Avg. B 1/4(Gate)
  Avg. B 2/1(Out) -> B2/1
  Gate 2/1 -> Avg. B 2/4(Gate)
  Reset/1 -> Avg. B 1/5(Reset), Avg. B 2/5(Reset)

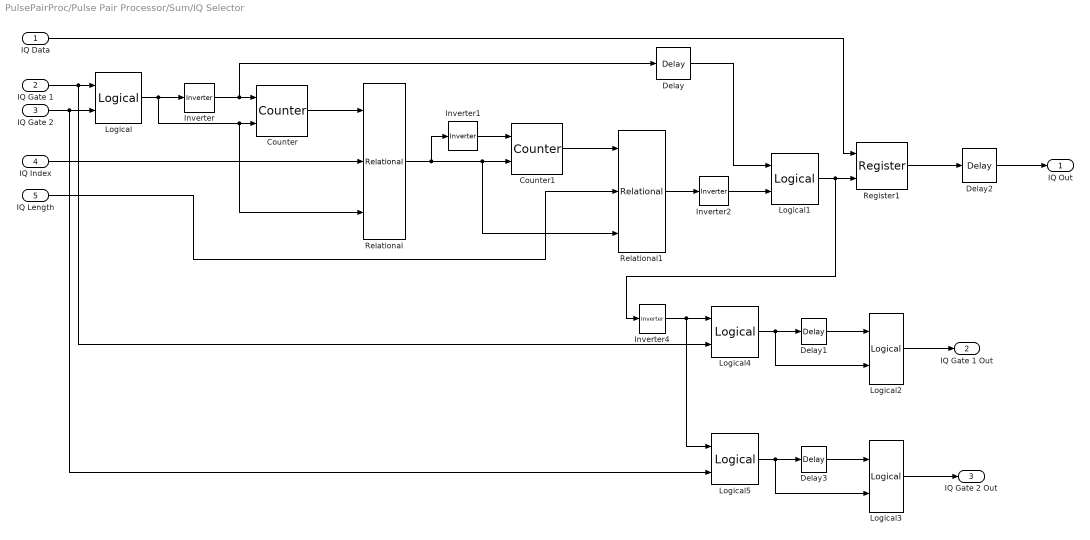
== system PulsePairProc/Pulse Pair Processor/Sum/IQ Selector ==
  IQ Data : Inport
  IQ Gate 1 : Inport  Port=2
  IQ Gate 2 : Inport  Port=3
  IQ Index : Inport  Port=4
  IQ Length : Inport  Port=5
  Counter : xbsIndex_r4/Counter  cnt_type=Count Limited  cnt_to=1023  operation=Up  start_count=0  cnt_by_val=1  arith_type=Unsigned  n_bits=10  bin_pt=0  load_pin=off  rst=on  en=on  explicit_period=on  period=1/12e6  dbl_ovrd=off  use_behavioral_HDL=off  use_rpm=off  block_type=counter
      settings: block_version=8.2
  Counter1 : xbsIndex_r4/Counter  cnt_type=Count Limited  cnt_to=1023  operation=Up  start_count=0  cnt_by_val=1  arith_type=Unsigned  n_bits=10  bin_pt=0  load_pin=off  rst=on  en=on  explicit_period=on  period=1/12e6  dbl_ovrd=off  use_behavioral_HDL=off  use_rpm=off  block_type=counter
      settings: block_version=8.2
  Delay{,1..3} (4 alike) : xbsIndex_r4/Delay  en=off  latency=3  dbl_ovrd=off  reg_retiming=off  block_type=delay
      settings: infoedit=Hardware notes: A delay line is a chain, each link of which is an SRL16 followed by a flip-flop. If register retiming is enabled, the delay line is a chain of flip-flops.  block_version=8.2
  Inverter : xbsIndex_r4/Inverter  en=off  latency=0  dbl_ovrd=off  block_type=inv
      settings: block_version=8.2
  Inverter1 : xbsIndex_r4/Inverter  en=off  latency=0  dbl_ovrd=off  block_type=inv
      settings: block_version=8.2
  Inverter2 : xbsIndex_r4/Inverter  en=off  latency=0  dbl_ovrd=off  block_type=inv
      settings: block_version=8.2
  Inverter4 : xbsIndex_r4/Inverter  en=off  latency=1  dbl_ovrd=off  block_type=inv
      settings: block_version=8.2
  Logical{,1..3} (4 alike) : xbsIndex_r4/Logical  logical_function=OR  inputs=2  en=off  latency=0  precision=Full  arith_type=Unsigned  n_bits=16  bin_pt=0  align_bp=on  dbl_ovrd=off  block_type=logical
      settings: block_version=8.2
  Logical4 : xbsIndex_r4/Logical  logical_function=AND  inputs=2  en=off  latency=0  precision=Full  arith_type=Unsigned  n_bits=16  bin_pt=0  align_bp=on  dbl_ovrd=off  block_type=logical
      settings: block_version=8.2
  Logical5 : xbsIndex_r4/Logical  logical_function=AND  inputs=2  en=off  latency=0  precision=Full  arith_type=Unsigned  n_bits=16  bin_pt=0  align_bp=on  dbl_ovrd=off  block_type=logical
      settings: block_version=8.2
  Register1 : xbsIndex_r4/Register  init=0  rst=on  en=off  dbl_ovrd=off  block_type=register
      settings: block_version=8.2
  Relational : xbsIndex_r4/Relational  mode=a>b  en=on  latency=1  dbl_ovrd=off  block_type=relational
      settings: block_version=8.2
  Relational1 : xbsIndex_r4/Relational  mode=a<b  en=on  latency=1  dbl_ovrd=off  block_type=relational
      settings: block_version=8.2
  IQ Out : Outport
  IQ Gate 1 Out : Outport  Port=2
  IQ Gate 2 Out : Outport  Port=3
  wires:
  Counter/1 -> Relational/1
  IQ Index/1 -> Relational/2
  Inverter/1 -> Counter/1, Delay/1
  Inverter1/1 -> Counter1/1
  Relational/1 -> Inverter1/1, Counter1/2, Relational1/3
  Counter1/1 -> Relational1/1
  Relational1/1 -> Inverter2/1
  IQ Data/1 -> Register1/1
  Register1/1 -> Delay2/1
  Logical/1 -> Inverter/1, Counter/2, Relational/3
  IQ Gate 2/1 -> Logical/2, Logical5/2
  IQ Gate 1/1 -> Logical/1, Logical4/2
  Logical1/1 -> Register1/2, Inverter4/1
  Inverter2/1 -> Logical1/2
  Delay/1 -> Logical1/1
  IQ Length/1 -> Relational1/2
  Logical2/1 -> IQ Gate 1 Out/1
  Delay1/1 -> Logical2/1
  Delay2/1 -> IQ Out/1
  Inverter4/1 -> Logical4/1, Logical5/1
  Logical4/1 -> Delay1/1, Logical2/2
  Logical3/1 -> IQ Gate 2 Out/1
  Delay3/1 -> Logical3/1
  Logical5/1 -> Delay3/1, Logical3/2

== system PulsePairProc/Pulse Pair Processor/Sum/P Avg ==
  P_Data_In : Inport
  M : Inport  Port=2
  N : Inport  Port=3
  Gate 1 : Inport  Port=4
  Gate 2 : Inport  Port=5
  Reset : Inport  Port=6
  Avg. P 1 : Subsystem
  Avg. P 2 : Subsystem
  P1 : Outport
  P2 : Outport  Port=2
  wires:
  P_Data_In/1 -> Avg. P 1/1(In), Avg. P 2/1(In)
  M/1 -> Avg. P 1/2(M), Avg. P 2/2(M)
  N/1 -> Avg. P 1/3(N), Avg. P 2/3(N)
  Avg. P 1/1(Out) -> P1/1
  Gate 1/1 -> Avg. P 1/4(Gate)
  Avg. P 2/1(Out) -> P2/1
  Gate 2/1 -> Avg. P 2/4(Gate)
  Reset/1 -> Avg. P 1/5(Reset), Avg. P 2/5(Reset)

== system PulsePairProc/Pulse Pair Processor/Calc/IQ_Delay/Wr Control ==
  Gate1 : Inport
  Gate2 : Inport  Port=2
  Constant : xbsIndex_r4/Constant  arith_type=Unsigned  const=0  n_bits=1  bin_pt=0  explicit_period=off  period=1  equ=P=C  opselect=C  inp2=PCIN>>17  opr=+  inp1=P  carry=CIN  dbl_ovrd=off  block_type=constant
      settings: block_version=8.2
  Convert : xbsIndex_r4/Convert  arith_type=Boolean  n_bits=16  bin_pt=14  quantization=Truncate  overflow=Wrap  latency=0  dbl_ovrd=off  pipeline=off  block_type=convert
      settings: block_version=8.2
  Convert1 : xbsIndex_r4/Convert  arith_type=Boolean  n_bits=16  bin_pt=14  quantization=Truncate  overflow=Wrap  latency=0  dbl_ovrd=off  pipeline=off  block_type=convert
      settings: block_version=8.2
  Counter : xbsIndex_r4/Counter  cnt_type=Free Running  cnt_to=Inf  operation=Up  start_count=0  cnt_by_val=1  arith_type=Unsigned  n_bits=11  bin_pt=0  load_pin=off  rst=on  en=on  explicit_period=off  period=1/12e6  dbl_ovrd=off  use_behavioral_HDL=off  use_rpm=off  block_type=counter
      settings: block_version=8.2
  Counter1 : xbsIndex_r4/Counter  cnt_type=Free Running  cnt_to=Inf  operation=Up  start_count=0  cnt_by_val=1  arith_type=Unsigned  n_bits=1  bin_pt=0  load_pin=off  rst=off  en=on  explicit_period=off  period=1/12e6  dbl_ovrd=off  use_behavioral_HDL=off  use_rpm=off  block_type=counter
      settings: block_version=8.2
  Delay1 : xbsIndex_r4/Delay  en=off  latency=1  dbl_ovrd=off  reg_retiming=off  block_type=delay
      settings: infoedit=Hardware notes: A delay line is a chain, each link of which is an SRL16 followed by a flip-flop. If register retiming is enabled, the delay line is a chain of flip-flops.  block_version=8.2
  Delay2 : xbsIndex_r4/Delay  en=off  latency=1  dbl_ovrd=off  reg_retiming=off  block_type=delay
      settings: infoedit=Hardware notes: A delay line is a chain, each link of which is an SRL16 followed by a flip-flop. If register retiming is enabled, the delay line is a chain of flip-flops.  block_version=8.2
  Inverter1 : xbsIndex_r4/Inverter  en=off  latency=0  dbl_ovrd=off  block_type=inv
      settings: block_version=8.2
  Inverter2 : xbsIndex_r4/Inverter  en=off  latency=0  dbl_ovrd=off  block_type=inv
      settings: block_version=8.2
  Logical : xbsIndex_r4/Logical  logical_function=OR  inputs=2  en=off  latency=0  precision=Full  arith_type=Unsigned  n_bits=16  bin_pt=0  align_bp=on  dbl_ovrd=off  block_type=logical
      settings: block_version=8.2
  Logical1 : xbsIndex_r4/Logical  logical_function=AND  inputs=2  en=off  latency=0  precision=Full  arith_type=Unsigned  n_bits=16  bin_pt=0  align_bp=on  dbl_ovrd=off  block_type=logical
      settings: block_version=8.2
  Register : xbsIndex_r4/Register  init=0  rst=on  en=on  dbl_ovrd=off  block_type=register
      settings: block_version=8.2
  Register1 : xbsIndex_r4/Register  init=0  rst=on  en=on  dbl_ovrd=off  block_type=register
      settings: block_version=8.2
  Relational1 : xbsIndex_r4/Relational  mode=a=b  en=off  latency=0  dbl_ovrd=off  block_type=relational
      settings: block_version=8.2
  Wr1 : Outport
  Wr2 : Outport  Port=2
  wires:
  Counter/1 -> Relational1/1
  Logical/1 -> Counter/2, Logical1/2, Delay1/1, Inverter2/1
  Inverter2/1 -> Counter/1, Delay2/1
  Counter1/1 -> Inverter1/1, Register/1
  Constant/1 -> Relational1/2
  Logical1/1 -> Counter1/1
  Relational1/1 -> Logical1/1
  Inverter1/1 -> Register1/1
  Delay1/1 -> Register1/3, Register/3
  Delay2/1 -> Register/2, Register1/2
  Gate1/1 -> Logical/1
  Gate2/1 -> Logical/2
  Register/1 -> Convert/1
  Register1/1 -> Convert1/1
  Convert/1 -> Wr1/1
  Convert1/1 -> Wr2/1

== system PulsePairProc/Pulse Pair Processor/Sum/A Avg/Avg. A 1 ==
  In : Inport
  M : Inport  Port=2
  N : Inport  Port=3
  Gate : Inport  Port=4
  Reset : Inport  Port=5
  AddSub1 : xbsIndex_r4/AddSub  mode=Addition  use_carryin=off  use_carryout=off  en=off  latency=0  precision=User Defined  arith_type="Signed  (2's comp)"  n_bits=33  bin_pt=31  quantization="Round  (unbiased: +/- Inf)"  overflow=Flag as error  dbl_ovrd=off  use_behavioral_HDL=off  pipelined=on  use_rpm=on  block_type=addsub
      settings: block_version=8.2
  Delay : xbsIndex_r4/Delay  en=off  latency=1  dbl_ovrd=off  reg_retiming=off  block_type=delay
      settings: infoedit=Hardware notes: A delay line is a chain, each link of which is an SRL16 followed by a flip-flop. If register retiming is enabled, the delay line is a chain of flip-flops.  block_version=8.2
  Delay1 : xbsIndex_r4/Delay  en=off  latency=1  dbl_ovrd=off  reg_retiming=off  block_type=delay
      settings: infoedit=Hardware notes: A delay line is a chain, each link of which is an SRL16 followed by a flip-flop. If register retiming is enabled, the delay line is a chain of flip-flops.  block_version=8.2
  FIFO : xbsIndex_r4/FIFO  depth=1K  percent_nbits=1  rst=on  en=off  dbl_ovrd=off  mem_type=Block RAM  block_type=fifo
      settings: block_version=8.2
  Logical : xbsIndex_r4/Logical  logical_function=OR  inputs=2  en=off  latency=0  precision=Full  arith_type=Unsigned  n_bits=16  bin_pt=0  align_bp=on  dbl_ovrd=off  block_type=logical
      settings: block_version=8.2
  Logical4 : xbsIndex_r4/Logical  logical_function=OR  inputs=2  en=off  latency=0  precision=Full  arith_type=Unsigned  n_bits=16  bin_pt=0  align_bp=on  dbl_ovrd=off  block_type=logical
      settings: block_version=8.2
  Mux : xbsIndex_r4/Mux  inputs=2  en=off  latency=0  precision=Full  arith_type=Unsigned  n_bits=16  bin_pt=14  quantization=Truncate  overflow=Wrap  dbl_ovrd=off  block_type=mux
      settings: block_version=8.2
  Register : xbsIndex_r4/Register  init=0  rst=on  en=on  dbl_ovrd=off  block_type=register
      settings: block_version=8.2
  Register1 : xbsIndex_r4/Register  init=0  rst=on  en=off  dbl_ovrd=off  block_type=register
      settings: block_version=8.2
  Shift : xbsIndex_r4/Shift  shift_dir=Right  shift_bits=1  en=off  latency=0  precision=User Defined  arith_type="Signed  (2's comp)"  n_bits=32  bin_pt=31  quantization="Round  (unbiased: +/- Inf)"  overflow=Flag as error  dbl_ovrd=off  block_type=shift
      settings: block_version=8.2
  Subsystem : Subsystem
  Out : Outport
  A,B,P Gate 1 : Outport  Port=2
  wires:
  Subsystem/1(WE) -> FIFO/2
  Subsystem/2(RE) -> Register1/1, FIFO/3
  Mux/1 -> FIFO/1, Register/1
  AddSub1/1 -> Shift/1
  FIFO/1 -> AddSub1/1
  Register1/1 -> Mux/1
  In/1 -> Delay/1
  Register/1 -> Out/1
  M/1 -> Subsystem/2(M)
  Subsystem/4(Out_En) -> Register/3, Delay1/1, Logical/2
  N/1 -> Subsystem/3(N)
  Delay/1 -> AddSub1/2, Mux/2
  Gate/1 -> Subsystem/1(Enable)
  Delay1/1 -> Logical/1
  Logical/1 -> A,B,P Gate 1/1
  Reset/1 -> Subsystem/4(Reset), Logical4/2, FIFO/4
  Logical4/1 -> Register1/2, Register/2
  Subsystem/3(RST) -> Logical4/1
  Shift/1 -> Mux/3
